simulink model "Bintang_Using_Vector"  (R2023a)
settings: Solver=VariableStepAuto  StartTime=0.0  StopTime=10.0  RelTol=1e-3
settings Model: Creator=Lenovo  LastModifiedBy=Lenovo

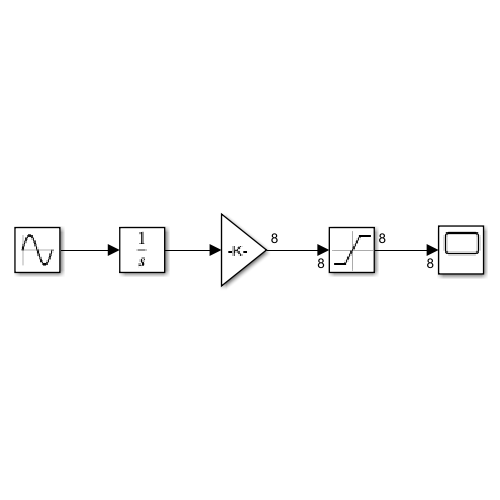
[thumbnail: Simulink's stored preview of the top-level diagram]
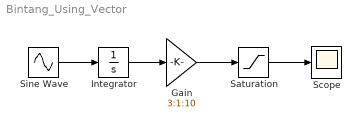
== system Bintang_Using_Vector ==
  Gain : Gain  Gain=3:1:10
  Integrator : Integrator
  Saturation : Saturate  UpperLimit=rand(8,1)*10  LowerLimit=rand(8,1)*.10
  Scope : Scope
  Sine Wave : Sin  SampleTime=0
  wires:
  Saturation/1 -> Scope/1
  Sine Wave/1 -> Integrator/1
  Integrator/1 -> Gain/1
  Gain/1 -> Saturation/1
